simulink model "model_robot_pendulum"  (R2017a)
settings: Solver=FixedStepAuto  StartTime=0.0  StopTime=30  FixedStep=1e-3  RelTol=1e-3
values from neighbouring files (symbols this model uses):
  phi_init = [phix_init, phiy_init]    [initialize_simulation.m]
libraries: sldrtlib x1
settings Model: Creator=Jan  LastModifiedBy=Jan

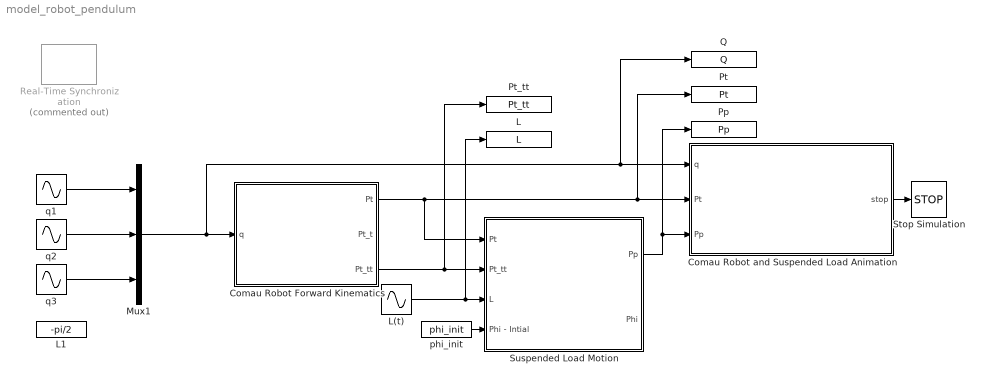
== system model_robot_pendulum ==
  Comau Robot Forward Kinematics : Subsystem
  Comau Robot and Suspended Load Animation : MATLAB Function  TreatAsAtomicUnit=on  SystemSampleTime=0.1
  L : ToWorkspace  VariableName=L  SampleTime=-1
      settings: Save2DSignal=2-D array (concatenate along first dimension)
  L(t) : Sin  Amplitude=0.5  Bias=2.0  Frequency=2*pi*0.05  SampleTime=0
  L1 : Constant  Value=-pi/2
  Mux1 : Mux  Inputs=3
  Pp : ToWorkspace  VariableName=Pp  SampleTime=-1
      settings: Save2DSignal=2-D array (concatenate along first dimension)
  Pt : ToWorkspace  VariableName=Pt  SampleTime=-1
  Pt_tt : ToWorkspace  VariableName=Pt_tt  SampleTime=-1
  Q : ToWorkspace  VariableName=Q  SampleTime=-1
      settings: Save2DSignal=2-D array (concatenate along first dimension)
  Real-Time Synchronization : sldrtlib/Real-Time Synchronization  Commented=on  SampleTime=0.1  MaxMissedTicks=10  ShowMissedTicks=off  YieldWhenWaiting=off
  Stop Simulation : Stop
  Suspended Load Motion : Subsystem
  phi_init : Constant  Value=phi_init
  q1 : Sin  Amplitude=30/180*pi  Frequency=2*pi*0.05  Phase=45/180*pi  SampleTime=0
  q2 : Sin  Amplitude=20/180*pi  Frequency=2*pi*0.1  Phase=90/180*pi  SampleTime=0
  q3 : Sin  Amplitude=15/180*pi  Bias=-pi/2  Frequency=2*pi*0.15  Phase=90/180*pi  SampleTime=0
  wires:
  q3/1 -> Mux1/3
  Comau Robot and Suspended Load Animation/1(stop) -> Stop Simulation/1
  L(t)/1 -> L/1, Suspended Load Motion/3(L)
  phi_init/1 -> Suspended Load Motion/4(Phi - Intial)
  Comau Robot Forward Kinematics/1(Pt) -> Pt/1, Comau Robot and Suspended Load Animation/2(Pt), Suspended Load Motion/1(Pt)
  Comau Robot Forward Kinematics/3(Pt_tt) -> Pt_tt/1, Suspended Load Motion/2(Pt_tt)
  Suspended Load Motion/1(Pp) -> Pp/1, Comau Robot and Suspended Load Animation/3(Pp)
  Mux1/1 -> Comau Robot Forward Kinematics/1(q), Q/1, Comau Robot and Suspended Load Animation/1(q)
  q1/1 -> Mux1/1
  q2/1 -> Mux1/2

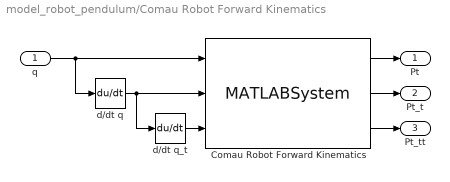
== system model_robot_pendulum/Comau Robot Forward Kinematics ==
  q : Inport
  Comau Robot Forward Kinematics : MATLABSystem  System=ComauRobotSystem  StringChoice=Forward Kinematics  SimulateUsing=Code generation
      mask Type: ComauRobotSystem
      mask Display:
      | disp('ComauRobotSystem');
      | port_label('input',1,'q');
      | port_label('input',2,'q_t');
      | port_label('input',3,'q_tt');
      | port_label('output',1,'P');
      | port_label('output',2,'P_t');
      | port_label('output',3,'P_tt');
  d/dt q : Derivative
  d/dt q_t : Derivative
  Pt : Outport
  Pt_t : Outport  Port=2
  Pt_tt : Outport  Port=3
  wires:
  d/dt q_t/1 -> Comau Robot Forward Kinematics/3
  d/dt q/1 -> Comau Robot Forward Kinematics/2, d/dt q_t/1
  Comau Robot Forward Kinematics/2 -> Pt_t/1
  q/1 -> d/dt q/1, Comau Robot Forward Kinematics/1
  Comau Robot Forward Kinematics/1 -> Pt/1
  Comau Robot Forward Kinematics/3 -> Pt_tt/1

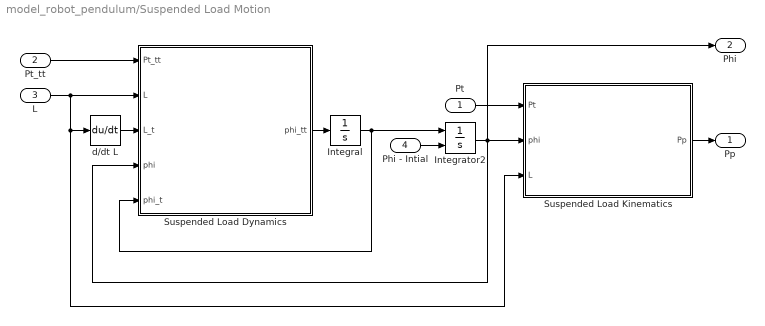
== system model_robot_pendulum/Suspended Load Motion ==
  Pt : Inport
  Pt_tt : Inport  Port=2
  L : Inport  Port=3
  Phi - Intial : Inport  Port=4
  Integral : Integrator  InitialCondition=[0 0]
  Integrator2 : Integrator  InitialConditionSource=external
  Suspended Load Dynamics : MATLAB Function  TreatAsAtomicUnit=on
  Suspended Load Kinematics : MATLAB Function  TreatAsAtomicUnit=on
  d/dt L : Derivative
  Pp : Outport
  Phi : Outport  Port=2
  wires:
  Pt/1 -> Suspended Load Kinematics/1(Pt)
  Suspended Load Dynamics/1(phi_tt) -> Integral/1
  Pt_tt/1 -> Suspended Load Dynamics/1(Pt_tt)
  L/1 -> Suspended Load Kinematics/3(L), d/dt L/1, Suspended Load Dynamics/2(L)
  Integral/1 -> Integrator2/1, Suspended Load Dynamics/5(phi_t)
  Integrator2/1 -> Phi/1, Suspended Load Kinematics/2(phi), Suspended Load Dynamics/4(phi)
  Phi - Intial/1 -> Integrator2/2
  Suspended Load Kinematics/1(Pp) -> Pp/1
  d/dt L/1 -> Suspended Load Dynamics/3(L_t)

== matlab function model_robot_pendulum/Comau Robot and Suspended Load Animation ==
  data: q input; stop output; Pt input; Pp input
function stop = SimulinkMotionPlot_ComauPendulum(q, Pt, Pp)
    % Creates a 3D-animation for the motion of the motion-lab system
    % Requires values for the Comau Robot joints and stewart platform
    % Input: 
    %	q	: Robot joint angular position
    %	Pt	: Tool-point position
    %	phi	: Pendulum Angular position euler angles
    % Output:
    %	stop :  Bool value to stop the anitmation
    
    % Persistent variables, to only be initialized once
    persistent h;           % Plot
    persistent Hr;          % Transformation Matrix
    stop = false;
    
    stop = false;
    
    %% Initialization 
    % One time intitialization of plotting settings
    if isempty(h)
        % Plotting setup
        h = figure('Name','StewartPlatform Animation');
        
        xlabel('x-axis')
        ylabel('y-axis')
        zlabel('z-axis')
        xlim([-2, 5])
        ylim([-2, 5])
        zlim([-2, 5])
        hold on;
        grid on;
        view(-30,20);
        
        % Reference coordinate system (world coordinate)
        Hr = eye(4);
    end
    
    %% Drawing
    if ishandle(h)
        cla;
        plot_robotpose(q, Hr); % Plot Robot pose
        plot_pendulum(Pt, Pp, Hr); % Plot Pendulum pose
        drawnow;
    end
    
    %% Destructor
    if ~ishandle(h)
        stop = true;
    end
end

%% Child functions

% Plot the pose of the Comau Robot
% This includes links and local coordinate systems
function plot_robotpose(q, Hr)
    % Inputs:
    % Hr : Transformation matrix of the robot base [4x4]
    % q  : Robot joints [3x1]
    
    % Static link lengths
    a1 = 0.350;
    a2 = 1.160;
    a3 = 0.250;
    d1 = 0.830;
    d4 = 1.4922;
    d6 = 0.210;
    dt = 0.567;
    L = d4 + d6 + dt;
    
    % Joint angles
    q1 = q(1);
    q2 = q(2);
    q3 = q(3);

    % Robot DH Table
    T1 = math3d.DH(-q1, d1, a1, pi/2);
    T2 = math3d.DH(pi/2 - q2, 0, a2, 0);
    T3 = math3d.DH(q3 + pi/2 + q2, 0, a3, pi/2);
    T4 = math3d.DH(pi, L, 0, 0);
            
    % Relative transformation
    Hr1 = Hr*T1;   % Robot base to joint q1 {r -> q1}
    Hr2 = Hr1*T2;   % Robot base to joint q2 {r -> q2}
    Hr3 = Hr2*T3;   % Robot base to joint q3 {r -> q2}
    Hr4 = Hr3*T4;   % Robot base to tool-point {r -> t}
    
    % Plot coordinate systems
    plot_coordinatesystem(Hr);      % Base
    plot_coordinatesystem(Hr1);     % Joint q1
    plot_coordinatesystem(Hr2);     % Joint q2
    plot_coordinatesystem(Hr3);     % Joint q3
    plot_coordinatesystem(Hr4);     % Tool-Point

    % Plot links
    plot_line(Hr(1:3,4), Hr1(1:3,4));	% Base to joint q1        
    plot_line(Hr1(1:3,4), Hr2(1:3,4));	% joint q1 to joint q2 
    plot_line(Hr2(1:3,4), Hr3(1:3,4));	% joint q2 to joint q3 
    plot_line(Hr3(1:3,4), Hr4(1:3,4));	% joint q3 to Tool-point
    
end

% Plot the position of the Pendulum
function plot_pendulum(Pt, Pp, Hr)
    % Inputs:
    % Pt    :   Tool-point position [3x]
    % Pp    :   Pendulum position [3x1]
    % Hr    :   Transformation matrix of the robot base [4x4]
    
    % Transforming the Position vector relative to world CSYS
    Pt = Hr*[Pt; 1];
    Pp = Hr*[Pp; 1];
    
    % Pendulum positions
    xp = Pp(1);
    yp = Pp(2);
    zp = Pp(3);
    
    % Plot wire
    plot_line(Pt(1:3), Pp(1:3));

    % Plot Load
    plot3(xp, yp, zp, 'ro', 'LineWidth', 5);
end
        
% Plot a line in 3D plots
function plot_line(p1, p2)
    % Inputs:
    %   p1  :   Point 1 [x1; y1; z1]
    %   p2  :   Point 2 [x2; y2; z2]

    % Pre-allocate
    line = zeros(2,3);

    line(1,:) = p1;
    line(2,:) = p2;

    X = line(:,1);
    Y = line(:,2);
    Z = line(:,3);

    plot3(X, Y, Z, 'k', 'LineWidth', 1)
end
        
% Plot the coordinate system in 3D plots
% with default rgb-colors to the related axis.
function plot_coordinatesystem(H)
    % Inputs:
    %   H       :   Transformation-matrix (size = 4x4)

    % Pre-allocate
    axis = zeros(2,3);
    
    % Rotation and Translation
    d = H(1:3,4);   % Translation vector
    R = H(1:3,1:3); % Rotation matrix

    % Axis colors
    colors = {'r', 'g', 'b'};
    
    % Length of each axis in csys
    csys_len = 0.5;
    
    % Plot all 3 axis
    % (Looping through plotting one axis at a time)
    for i = 1:3
        axis(1,:) = d;                      % csys origo [x0 y0 z0]
        axis(2,:) = d + R(:,i)*csys_len;    % end point of axis [x y z]

        X = axis(:,1);  % Vector of the x-component
        Y = axis(:,2);  % Vector of the y-component
        Z = axis(:,3);  % Vector of the z-component

        % Plot one of the axis with the related color
        plot3(X, Y, Z, colors{i}, 'LineWidth', 1)
    end
end

== matlab function model_robot_pendulum/Suspended Load Motion/Suspended Load Dynamics ==
  data: Pt_tt input; L input; L_t input; phi_tt output; phi input; phi_t input
function phi_tt = pendulumDynamics(Pt_tt, L, L_t, phi, phi_t)
    % Calculates the dynamics of the suspended load
    % Derives the differential equation for the euler angles
    %
    % Input: 
    %	Pt_tt   : Tool-point acceleration
    %	phi     : Pendulum Angular position euler angles
    %   phit_t  : Pendulum Angular velocity euler angles
    %   L       : Wire length
    %   L_t     : Wire velocity
    %
    %   Output  :
    %   phit_t  : Pendulum Angular acceleration euler angles
    
    % Parameters
    g = 9.81;   % Gravity
    
    % Tool-point acceleration components
    xt_tt = Pt_tt(1); 
    yt_tt = Pt_tt(2); 
    zt_tt = Pt_tt(3);

    % Pendulum euler angles (angular position)
    phix = phi(1);
    phiy = phi(2);

    % Pendulum euler angles (angular velocity)
    phix_t = phi_t(1);
    phiy_t = phi_t(2);
    
     % Pendulum ODE of the euler angles
    % (found from euler-lagrange equation,
    %  derived by the use of Maple)
    phix_tt = (xt_tt*cos(phix) + yt_tt*sin(phix)*sin(phiy) ...
              - zt_tt*sin(phix)*cos(phiy) ...
              - g*sin(phix)*cos(phiy) ...
              - 2*L_t*phix_t ...
              - L*phiy_t^2*sin(phix)*cos(phix)) / L;

    phiy_tt = (- yt_tt*cos(phiy) - zt_tt*sin(phiy) ...
              - g*sin(phiy) + 2*L_t*phiy_t*cos(phix) ...
              + 2*L*phix_t*phiy_t*sin(phix)) ...
              / (L*cos(phix));

    phi_tt = [phix_tt; phiy_tt];

== matlab function model_robot_pendulum/Suspended Load Motion/Suspended Load Kinematics ==
  data: Pt input; phi input; L input; Pp output
function Pp = pendulumKinematics(Pt, phi, L)
    % Calculates the kinematics of the suspended load
    
    % Input: 
    %	Pt_tt   : Tool-point position
    %	phi     : Pendulum Angular position euler angles
    %   L       : Wire length
    
    
    % Tool-point position 
    xt = Pt(1);
    yt = Pt(2);
    zt = Pt(3);

    % Pendulum euler angles
    phix = phi(1);
    phiy = phi(2);

    % Pendulum position 
    xp = xt - L*sin(phix);
    yp = yt + L*cos(phix)*sin(phiy);
    zp = zt - L*cos(phix)*cos(phiy);

    Pp = [xp; yp; zp];
end
